simulink model "Ref"  (R2024b)
settings: Solver=VariableStepAuto  StartTime=0.0  StopTime=10.0  RelTol=1e-3
undefined symbols (not defined in the file or in its folder): env, IC, orb
settings Model: Creator=parrot  LastModifiedBy=parrot

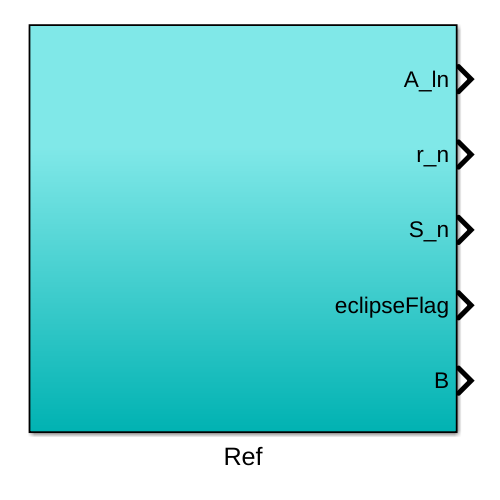
[thumbnail: Simulink's stored preview of the top-level diagram]
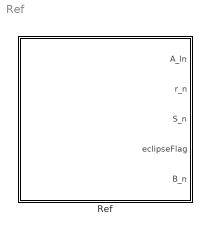
== system Ref ==
  Ref : Subsystem

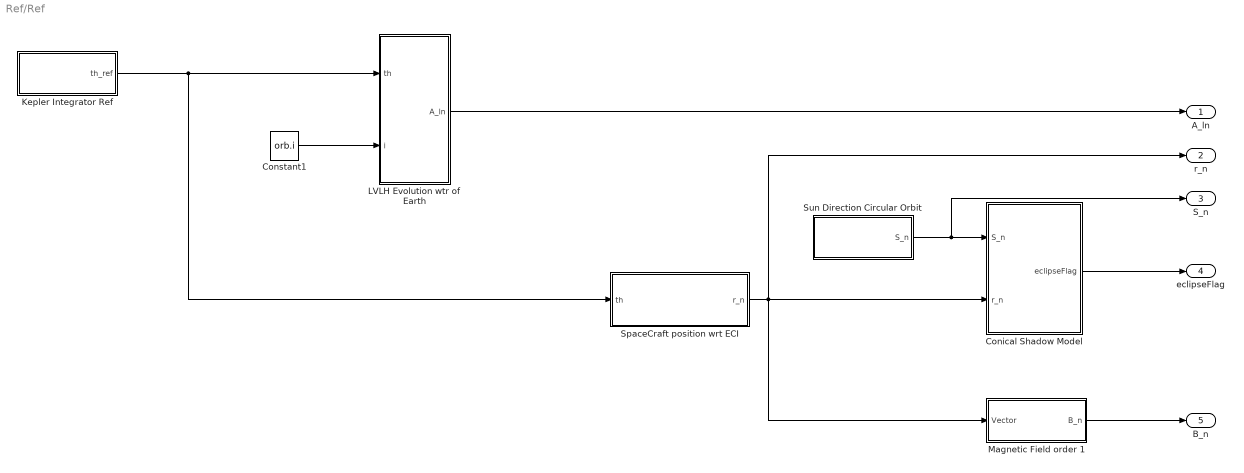
== system Ref/Ref ==
  Conical Shadow Model : Subsystem
  Constant1 : Constant  Value=orb.i
  Kepler Integrator Ref : Subsystem
  LVLH Evolution wtr of Earth : Subsystem
  Magnetic Field order 1 : Subsystem
  SpaceCraft position wrt ECI : Subsystem
  Sun Direction Circular Orbit : Subsystem
  A_ln : Outport
  r_n : Outport  Port=2
  S_n : Outport  Port=3
  eclipseFlag : Outport  Port=4
  B_n : Outport  Port=5
  wires:
  Kepler Integrator Ref/1(th_ref) -> SpaceCraft position wrt ECI/1(th), LVLH Evolution wtr of Earth/1(th)
  Constant1/1 -> LVLH Evolution wtr of Earth/2(i)
  LVLH Evolution wtr of Earth/1(A_ln) -> A_ln/1
  Sun Direction Circular Orbit/1(S_n) -> S_n/1, Conical Shadow Model/1(S_n)
  SpaceCraft position wrt ECI/1(r_n) -> Magnetic Field order 1/1(Vector), r_n/1, Conical Shadow Model/2(r_n)
  Conical Shadow Model/1(eclipseFlag) -> eclipseFlag/1
  Magnetic Field order 1/1(B_n) -> B_n/1

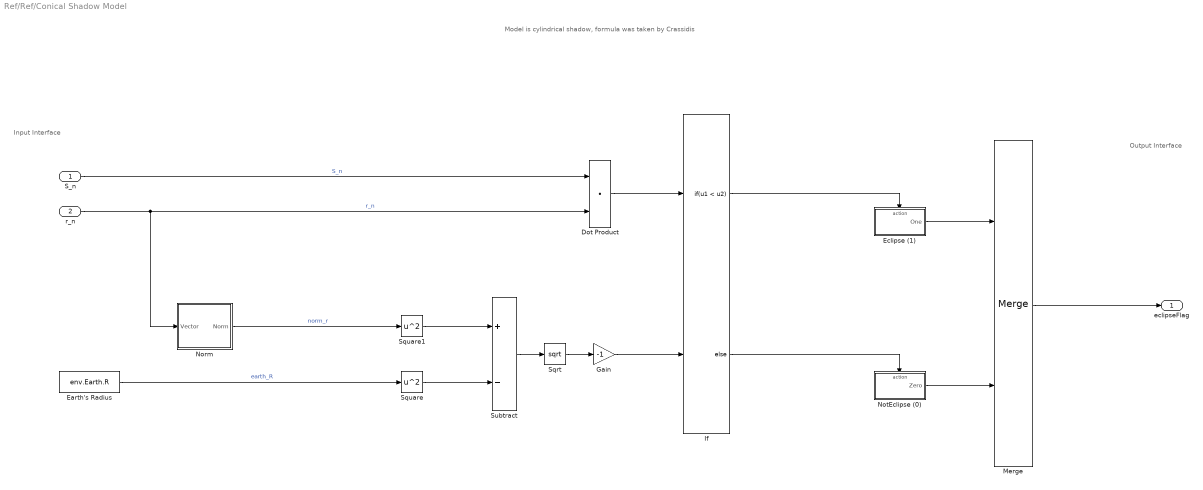
== system Ref/Ref/Conical Shadow Model ==
  note: Output Interface
  note: Input Interface
  note: Model is cylindrical shadow, formula was taken by Crassidis
  S_n : Inport
  r_n : Inport  Port=2
  Dot Product : DotProduct  OutDataTypeStr=Inherit: Inherit via internal rule
  Earth's Radius : Constant  Value=env.Earth.R
  Eclipse (1) : Subsystem  TreatAsAtomicUnit=on
  Gain : Gain  Gain=-1
  If : If  NumInputs=2  IfExpression=u1 < u2
  Merge : Merge
  Norm : Subsystem
  NotEclipse (0) : Subsystem  TreatAsAtomicUnit=on
  Sqrt : Sqrt
  Square : Math  Operator=square
  Square1 : Math  Operator=square
  Subtract : Sum  Inputs=+-
  eclipseFlag : Outport
  wires:
  r_n/1 -> Dot Product/2, Norm/1(Vector)  "r_n"
  S_n/1 -> Dot Product/1  "S_n"
  Norm/1(Norm) -> Square1/1  "norm_r"
  If/1 -> Eclipse (1)/Action
  If/2 -> NotEclipse (0)/Action
  Merge/1 -> eclipseFlag/1
  Eclipse (1)/1(One) -> Merge/1
  NotEclipse (0)/1(Zero) -> Merge/2
  Dot Product/1 -> If/1
  Gain/1 -> If/2
  Sqrt/1 -> Gain/1
  Subtract/1 -> Sqrt/1
  Square/1 -> Subtract/2
  Square1/1 -> Subtract/1
  Earth's Radius/1 -> Square/1  "earth_R"

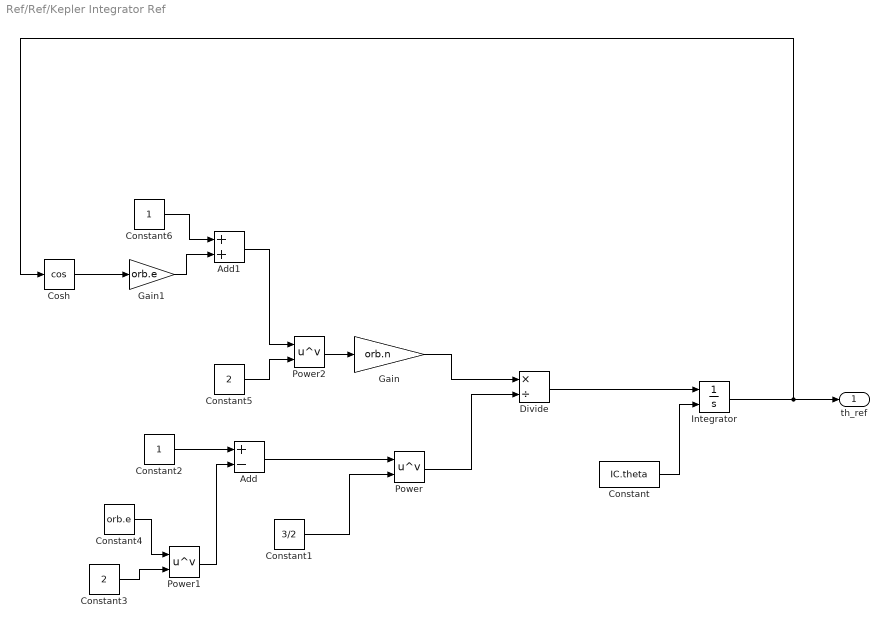
== system Ref/Ref/Kepler Integrator Ref ==
  Add : Sum  Inputs=+-
  Add1 : Sum
  Constant : Constant  Value=IC.theta
  Constant1 : Constant  Value=3/2
  Constant2 : Constant
  Constant3 : Constant  Value=2
  Constant4 : Constant  Value=orb.e
  Constant5 : Constant  Value=2
  Constant6 : Constant
  Cosh : Trigonometry  Operator=cos
  Divide : Product  Inputs=*/
  Gain : Gain  Gain=orb.n
  Gain1 : Gain  Gain=orb.e
  Integrator : Integrator  InitialConditionSource=external  WrapState=on  WrappedStateUpperValue=2*pi  WrappedStateLowerValue=0
  Power : Math  Operator=pow
  Power1 : Math  Operator=pow
  Power2 : Math  Operator=pow
  th_ref : Outport
  wires:
  Constant/1 -> Integrator/2
  Integrator/1 -> Cosh/1, th_ref/1
  Divide/1 -> Integrator/1
  Power/1 -> Divide/2
  Constant1/1 -> Power/2
  Constant2/1 -> Add/1
  Add/1 -> Power/1
  Power1/1 -> Add/2
  Constant3/1 -> Power1/2
  Constant4/1 -> Power1/1
  Gain/1 -> Divide/1
  Power2/1 -> Gain/1
  Constant5/1 -> Power2/2
  Add1/1 -> Power2/1
  Constant6/1 -> Add1/1
  Gain1/1 -> Add1/2
  Cosh/1 -> Gain1/1

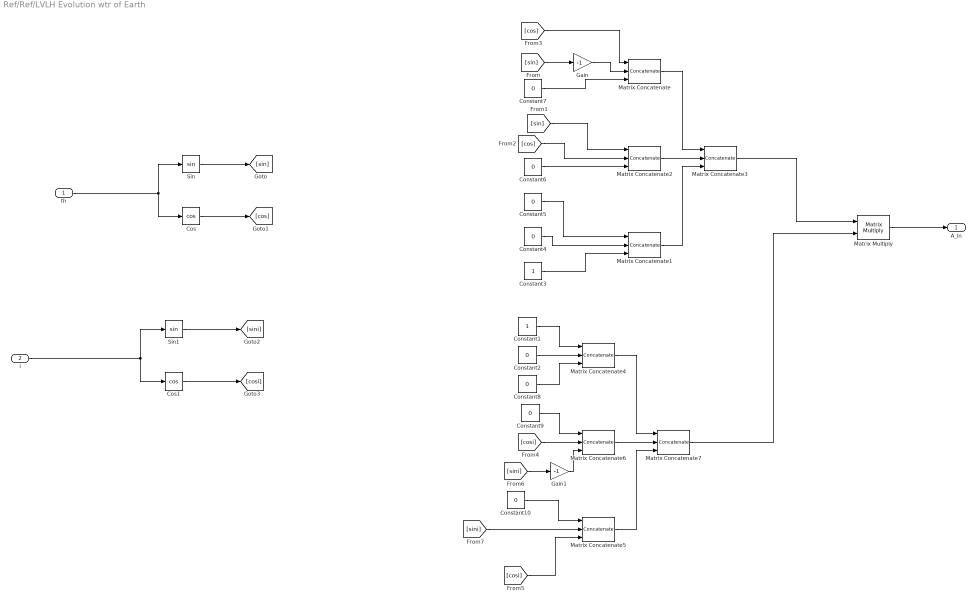
== system Ref/Ref/LVLH Evolution wtr of Earth ==
  th : Inport
  i : Inport  Port=2
  Constant1 : Constant
  Constant{2,4..10} (8 alike) : Constant  Value=0
  Constant3 : Constant
  Cos : Trigonometry  Operator=cos
  Cos1 : Trigonometry  Operator=cos
  Gain : Gain  Gain=-1
  Gain1 : Gain  Gain=-1
  Matrix Concatenate{,1..2,4..6} (6 alike) : Concatenate  NumInputs=3  Mode=Multidimensional array
  Matrix Concatenate3 : Concatenate  NumInputs=3  Mode=Multidimensional array  ConcatenateDimension=2
  Matrix Concatenate7 : Concatenate  NumInputs=3  Mode=Multidimensional array  ConcatenateDimension=2
  Matrix Multiply : Product  Multiplication=Matrix(*)
  Sin : Trigonometry
  Sin1 : Trigonometry
  A_ln : Outport
  wires:
  Cos/1 -> [cos]
  Matrix Concatenate1/1 -> Matrix Concatenate3/3
  th/1 -> Cos/1, Sin/1
  Matrix Concatenate/1 -> Matrix Concatenate3/1
  Constant5/1 -> Matrix Concatenate1/1
  Constant3/1 -> Matrix Concatenate1/3
  [cos] -> Matrix Concatenate/1
  Sin/1 -> [sin]
  Constant6/1 -> Matrix Concatenate2/3
  Constant7/1 -> Matrix Concatenate/3
  Constant4/1 -> Matrix Concatenate1/2
  Matrix Concatenate2/1 -> Matrix Concatenate3/2
  [cos] -> Matrix Concatenate2/2
  [sin] -> Matrix Concatenate2/1
  Gain/1 -> Matrix Concatenate/2
  [sin] -> Gain/1
  Cos1/1 -> [cosi]
  Sin1/1 -> [sini]
  i/1 -> Cos1/1, Sin1/1
  Matrix Multiply/1 -> A_ln/1
  Matrix Concatenate3/1 -> Matrix Multiply/1
  Matrix Concatenate7/1 -> Matrix Multiply/2
  Matrix Concatenate6/1 -> Matrix Concatenate7/2
  Matrix Concatenate5/1 -> Matrix Concatenate7/3
  Matrix Concatenate4/1 -> Matrix Concatenate7/1
  Constant1/1 -> Matrix Concatenate4/1
  Constant2/1 -> Matrix Concatenate4/2
  Constant8/1 -> Matrix Concatenate4/3
  Constant9/1 -> Matrix Concatenate6/1
  Constant10/1 -> Matrix Concatenate5/1
  [cosi] -> Matrix Concatenate5/3
  [cosi] -> Matrix Concatenate6/2
  [sini] -> Matrix Concatenate5/2
  [sini] -> Gain1/1
  Gain1/1 -> Matrix Concatenate6/3

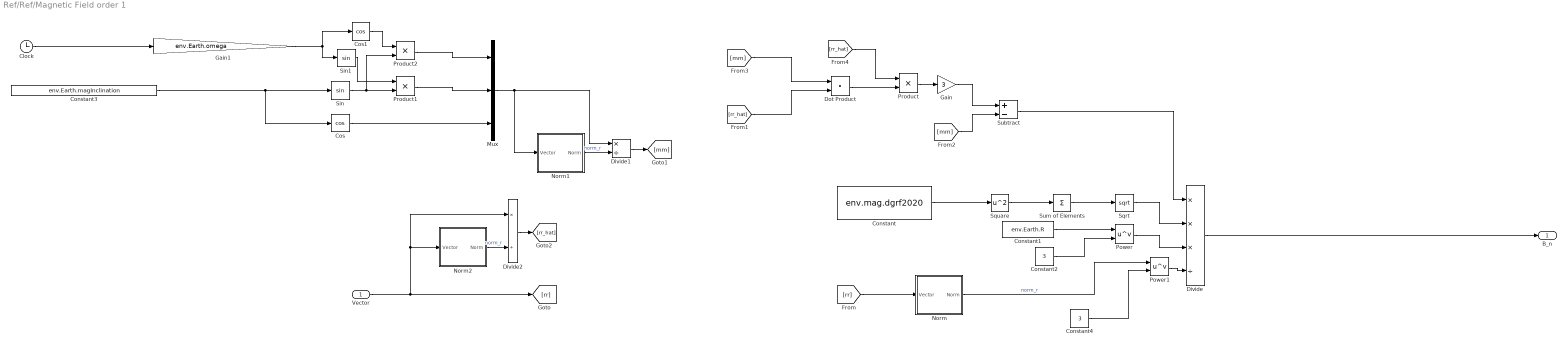
== system Ref/Ref/Magnetic Field order 1 ==
  Vector : Inport
  Clock : Clock
  Constant : Constant  Value=env.mag.dgrf2020
  Constant1 : Constant  Value=env.Earth.R
  Constant2 : Constant  Value=3
  Constant3 : Constant  Value=env.Earth.magInclination
  Constant4 : Constant  Value=3
  Cos : Trigonometry  Operator=cos
  Cos1 : Trigonometry  Operator=cos
  Divide : Product  Inputs=***/
  Divide1 : Product  Inputs=*/
  Divide2 : Product  Inputs=*/
  Dot Product : DotProduct  OutDataTypeStr=Inherit: Inherit via internal rule
  Gain : Gain  Gain=3
  Gain1 : Gain  Gain=env.Earth.omega
  Mux : Mux  Inputs=3
  Norm : Subsystem
  Norm1 : Subsystem
  Norm2 : Subsystem
  Power : Math  Operator=pow
  Power1 : Math  Operator=pow
  Product : Product
  Product1 : Product
  Product2 : Product
  Sin : Trigonometry
  Sin1 : Trigonometry
  Sqrt : Sqrt
  Square : Math  Operator=square
  Subtract : Sum  Inputs=+-
  Sum of Elements : Sum  Inputs=+
  B_n : Outport
  wires:
  Constant/1 -> Square/1
  Square/1 -> Sum of Elements/1
  Sum of Elements/1 -> Sqrt/1
  Constant1/1 -> Power/1
  Constant2/1 -> Power/2
  Sqrt/1 -> Divide/2
  Power/1 -> Divide/3
  Constant4/1 -> Power1/2
  Power1/1 -> Divide/4
  Norm/1(Norm) -> Power1/1  "norm_r"
  Vector/1 -> Norm2/1(Vector), Divide2/1, [rr]
  [rr] -> Norm/1(Vector)
  [rr_hat] -> Dot Product/2
  Subtract/1 -> Divide/1
  [mm] -> Subtract/2
  Dot Product/1 -> Product/2
  Product/1 -> Gain/1
  Gain/1 -> Subtract/1
  [rr_hat] -> Product/1
  [mm] -> Dot Product/1
  Mux/1 -> Norm1/1(Vector), Divide1/1
  Cos/1 -> Mux/3
  Constant3/1 -> Sin/1, Cos/1
  Clock/1 -> Gain1/1
  Sin/1 -> Product2/2, Product1/2
  Product1/1 -> Mux/2
  Product2/1 -> Mux/1
  Cos1/1 -> Product2/1
  Gain1/1 -> Cos1/1, Sin1/1
  Sin1/1 -> Product1/1
  Divide/1 -> B_n/1
  Norm1/1(Norm) -> Divide1/2  "norm_r"
  Divide1/1 -> [mm]
  Norm2/1(Norm) -> Divide2/2  "norm_r"
  Divide2/1 -> [rr_hat]

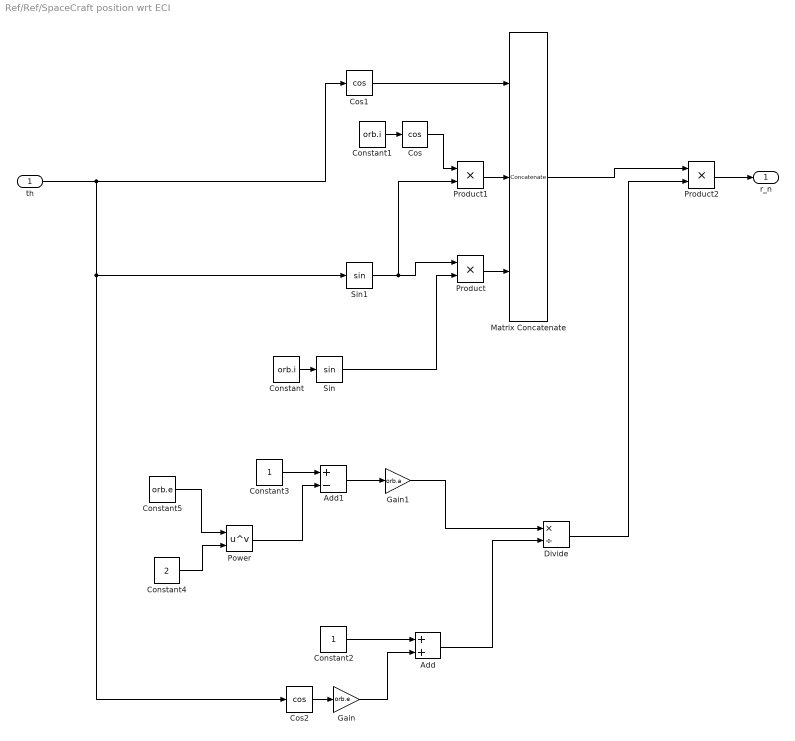
== system Ref/Ref/SpaceCraft position wrt ECI ==
  th : Inport
  Add : Sum
  Add1 : Sum  Inputs=+-
  Constant : Constant  Value=orb.i
  Constant1 : Constant  Value=orb.i
  Constant2 : Constant
  Constant3 : Constant
  Constant4 : Constant  Value=2
  Constant5 : Constant  Value=orb.e
  Cos : Trigonometry  Operator=cos
  Cos1 : Trigonometry  Operator=cos
  Cos2 : Trigonometry  Operator=cos
  Divide : Product  Inputs=*/
  Gain : Gain  Gain=orb.e
  Gain1 : Gain  Gain=orb.a
  Matrix Concatenate : Concatenate  NumInputs=3  Mode=Multidimensional array
  Power : Math  Operator=pow
  Product : Product
  Product1 : Product
  Product2 : Product
  Sin : Trigonometry
  Sin1 : Trigonometry
  r_n : Outport
  wires:
  Constant/1 -> Sin/1
  Cos1/1 -> Matrix Concatenate/1
  th/1 -> Sin1/1, Cos2/1, Cos1/1
  Product1/1 -> Matrix Concatenate/2
  Product/1 -> Matrix Concatenate/3
  Sin1/1 -> Product1/2, Product/1
  Sin/1 -> Product/2
  Constant1/1 -> Cos/1
  Cos/1 -> Product1/1
  Product2/1 -> r_n/1
  Matrix Concatenate/1 -> Product2/1
  Divide/1 -> Product2/2
  Constant2/1 -> Add/1
  Add/1 -> Divide/2
  Cos2/1 -> Gain/1
  Gain/1 -> Add/2
  Constant3/1 -> Add1/1
  Power/1 -> Add1/2
  Constant4/1 -> Power/2
  Constant5/1 -> Power/1
  Add1/1 -> Gain1/1
  Gain1/1 -> Divide/1

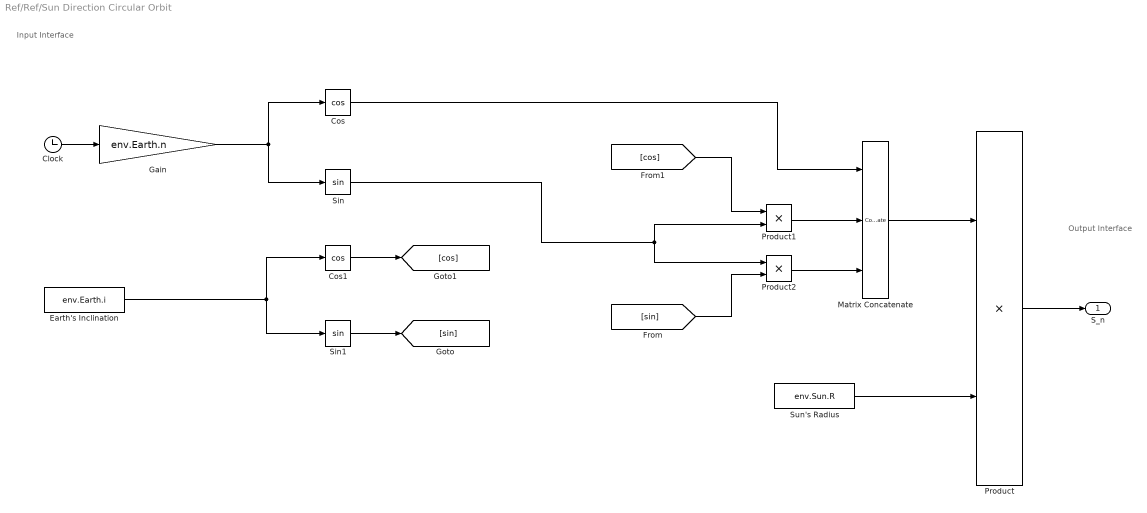
== system Ref/Ref/Sun Direction Circular Orbit ==
  note: Input Interface
  note: Output Interface
  Clock : Clock
  Cos : Trigonometry  Operator=cos
  Cos1 : Trigonometry  Operator=cos
  Earth's Inclination : Constant  Value=env.Earth.i
  Gain : Gain  Gain=env.Earth.n
  Matrix Concatenate : Concatenate  NumInputs=3  Mode=Multidimensional array
  Product : Product
  Product1 : Product
  Product2 : Product
  Sin : Trigonometry
  Sin1 : Trigonometry
  Sun's Radius : Constant  Value=env.Sun.R
  S_n : Outport
  wires:
  Clock/1 -> Gain/1
  Gain/1 -> Sin/1, Cos/1
  Product/1 -> S_n/1
  Sun's Radius/1 -> Product/2
  Matrix Concatenate/1 -> Product/1
  Earth's Inclination/1 -> Sin1/1, Cos1/1
  Cos1/1 -> [cos]
  Sin1/1 -> [sin]
  Cos/1 -> Matrix Concatenate/1
  Product1/1 -> Matrix Concatenate/2
  Product2/1 -> Matrix Concatenate/3
  [sin] -> Product2/2
  [cos] -> Product1/1
  Sin/1 -> Product1/2, Product2/1

== system Ref/Ref/Conical Shadow Model/Eclipse (1) ==
  Action Port : ActionPort
  Constant : Constant
  One : Outport
  wires:
  Constant/1 -> One/1

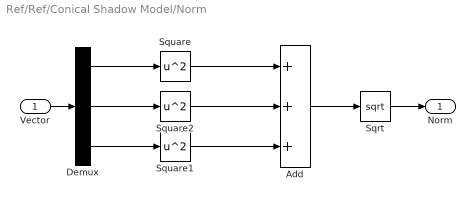
== system Ref/Ref/Conical Shadow Model/Norm ==
  Vector : Inport
  Add : Sum  Inputs=+++
  Demux : Demux  Outputs=3
  Sqrt : Sqrt
  Square : Math  Operator=square
  Square1 : Math  Operator=square
  Square2 : Math  Operator=square
  Norm : Outport
  wires:
  Square/1 -> Add/1
  Add/1 -> Sqrt/1
  Demux/3 -> Square1/1
  Square2/1 -> Add/2
  Square1/1 -> Add/3
  Demux/1 -> Square/1
  Demux/2 -> Square2/1
  Vector/1 -> Demux/1
  Sqrt/1 -> Norm/1

== system Ref/Ref/Conical Shadow Model/NotEclipse (0) ==
  Action Port : ActionPort
  Constant : Constant  Value=0
  Zero : Outport
  wires:
  Constant/1 -> Zero/1

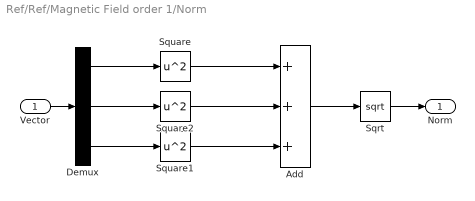
== system Ref/Ref/Magnetic Field order 1/Norm ==
  Vector : Inport
  Add : Sum  Inputs=+++
  Demux : Demux  Outputs=3
  Sqrt : Sqrt
  Square : Math  Operator=square
  Square1 : Math  Operator=square
  Square2 : Math  Operator=square
  Norm : Outport
  wires:
  Square/1 -> Add/1
  Add/1 -> Sqrt/1
  Demux/3 -> Square1/1
  Square2/1 -> Add/2
  Square1/1 -> Add/3
  Demux/1 -> Square/1
  Demux/2 -> Square2/1
  Vector/1 -> Demux/1
  Sqrt/1 -> Norm/1

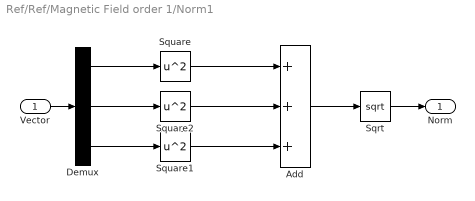
== system Ref/Ref/Magnetic Field order 1/Norm1 ==
  Vector : Inport
  Add : Sum  Inputs=+++
  Demux : Demux  Outputs=3
  Sqrt : Sqrt
  Square : Math  Operator=square
  Square1 : Math  Operator=square
  Square2 : Math  Operator=square
  Norm : Outport
  wires:
  Square/1 -> Add/1
  Add/1 -> Sqrt/1
  Demux/3 -> Square1/1
  Square2/1 -> Add/2
  Square1/1 -> Add/3
  Demux/1 -> Square/1
  Demux/2 -> Square2/1
  Vector/1 -> Demux/1
  Sqrt/1 -> Norm/1

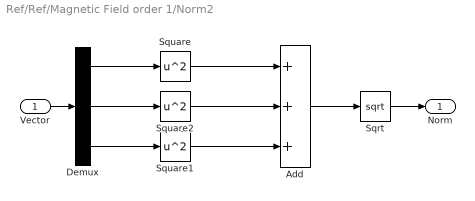
== system Ref/Ref/Magnetic Field order 1/Norm2 ==
  Vector : Inport
  Add : Sum  Inputs=+++
  Demux : Demux  Outputs=3
  Sqrt : Sqrt
  Square : Math  Operator=square
  Square1 : Math  Operator=square
  Square2 : Math  Operator=square
  Norm : Outport
  wires:
  Square/1 -> Add/1
  Add/1 -> Sqrt/1
  Demux/3 -> Square1/1
  Square2/1 -> Add/2
  Square1/1 -> Add/3
  Demux/1 -> Square/1
  Demux/2 -> Square2/1
  Vector/1 -> Demux/1
  Sqrt/1 -> Norm/1
